simulink model "model31"  (R2024a)
settings: Solver=VariableStepAuto  StartTime=0.0  StopTime=10  MaxStep=1e-3  RelTol=1e-3
values from neighbouring files (symbols this model uses):
  A = [8 1 11 ... (first row only)    [init.m]    (also in init_ex.m)
  B = [-1; -3; 3]    [init.m]    (also in init_ex.m)
  B_f = [1, -1 ... (first row only)    [init.m]    (also in init_ex.m)
  C = [-2 0 -3]    [init.m]    (also in init_ex.m)
  C_st = [0  0 -1 ... (first row only)    [init.m]
  D = 15    [init.m]    (also in init_ex.m)
  D_f = [0 3]    [init.m]    (also in init_ex.m)
  F = G_f - L_st * Y_f    [init.m]
  G = [-5 0 0 ... (first row only)    [init.m]    (also in init_ex.m)
  G_f = [35 10 -28 17 ... (first row only)    [init.m]    (also in init_ex.m)
  G_g = [0 0 0 ... (first row only)    [init.m]    (also in init_ex.m)
  K = [-3.5 1 -3.5]    [init.m]    (also in init_ex.m)
  K_f = [-9.2262   -2.9556    6.9958   -4.9150]    [init.m]    (also in init_ex.m)
  K_g = [0.0703   -0.0562    0.0658]    [init.m]    (also in init_ex.m)
  L_st = -(Y_st * inv(Q_st))'    [init.m]
  Q_inv = inv(Q)    [init.m]    (also in init_ex.m)
  wf0 = [1; 1; 1; 1]    [init.m]    (also in init_ex.m)
  wg0 = [-12; 0; 21]    [init.m]    (also in init_ex.m)
  x0 = [0; 0; 0]    [init.m]    (also in init_ex.m)
  Y = [1; 7; 8]    [init.m]    (also in init_ex.m)
  Y_f = [12 -6 ... (first row only)    [init.m]    (also in init_ex.m)
  Y_g = [1, 1, 0]    [init.m]    (also in init_ex.m)
settings Model: Creator=eva  LastModifiedBy=eva

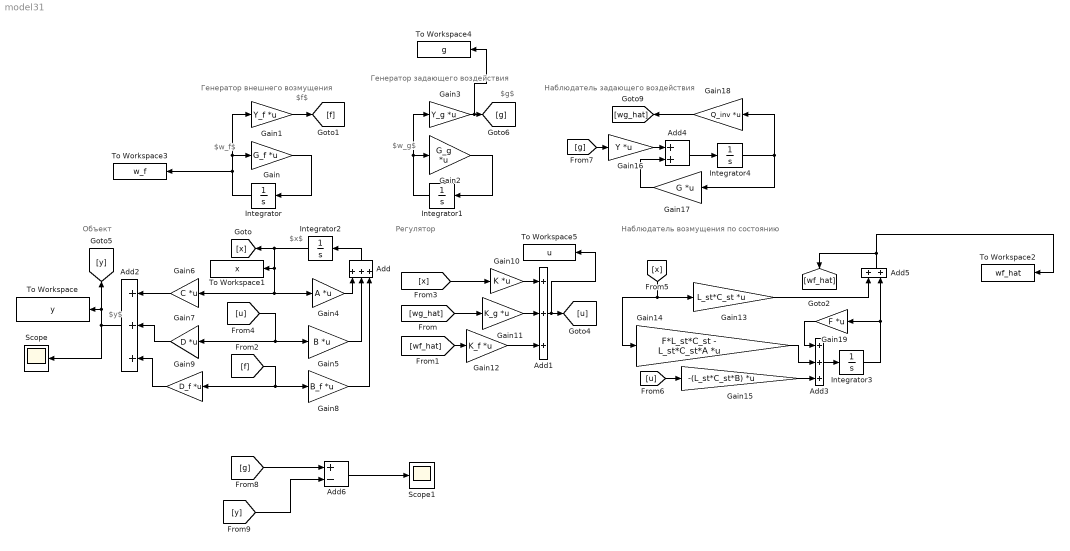
== system model31 ==
  note: Наблюдатель возмущения по состоянию
  note: Объект
  note: Наблюдатель задающего воздействия
  note: $y$
  note: $x$
  note: Регулятор
  note: $g$
  note: $w_f$
  note: Генератор задающего воздействия
  note: $w_g$
  note: $f$
  note: Генератор внешнего возмущения
  Add{,1..3} (4 alike) : Sum  Inputs=+++
  Add4 : Sum
  Add5 : Sum
  Add6 : Sum  Inputs=+-
  Gain : Gain  Gain=G_f  Multiplication=Matrix(K*u)
  Gain1 : Gain  Gain=Y_f  Multiplication=Matrix(K*u)
  Gain10 : Gain  Gain=K  Multiplication=Matrix(K*u)
  Gain11 : Gain  Gain=K_g  Multiplication=Matrix(K*u)
  Gain12 : Gain  Gain=K_f  Multiplication=Matrix(K*u)
  Gain13 : Gain  Gain=L_st*C_st  Multiplication=Matrix(K*u)
  Gain14 : Gain  Gain=F*L_st*C_st - L_st*C_st*A  Multiplication=Matrix(K*u)
  Gain15 : Gain  Gain=-(L_st*C_st*B)  Multiplication=Matrix(K*u)
  Gain16 : Gain  Gain=Y  Multiplication=Matrix(K*u)
  Gain17 : Gain  Gain=G  Multiplication=Matrix(K*u)
  Gain18 : Gain  Gain=Q_inv  Multiplication=Matrix(K*u)
  Gain19 : Gain  Gain=F  Multiplication=Matrix(K*u)
  Gain2 : Gain  Gain=G_g  Multiplication=Matrix(K*u)
  Gain3 : Gain  Gain=Y_g  Multiplication=Matrix(K*u)
  Gain4 : Gain  Gain=A  Multiplication=Matrix(K*u)
  Gain5 : Gain  Gain=B  Multiplication=Matrix(K*u)
  Gain6 : Gain  Gain=C  Multiplication=Matrix(K*u)
  Gain7 : Gain  Gain=D  Multiplication=Matrix(K*u)
  Gain8 : Gain  Gain=B_f  Multiplication=Matrix(K*u)
  Gain9 : Gain  Gain=D_f  Multiplication=Matrix(K*u)
  Integrator : Integrator  InitialCondition=wf0
  Integrator1 : Integrator  InitialCondition=wg0
  Integrator2 : Integrator  InitialCondition=x0
  Integrator3 : Integrator  InitialCondition=[0; 0; 0; 0]
  Integrator4 : Integrator  InitialCondition=[0; 0; 0]
  Scope : Scope
  Scope1 : Scope
  To Workspace : ToWorkspace  VariableName=y  SaveFormat=Structure With Time  SampleTime=-1
  To Workspace1 : ToWorkspace  VariableName=x  SaveFormat=Structure With Time  SampleTime=-1
  To Workspace2 : ToWorkspace  VariableName=wf_hat  SaveFormat=Structure With Time  SampleTime=-1
  To Workspace3 : ToWorkspace  VariableName=w_f  SaveFormat=Structure With Time  SampleTime=-1
  To Workspace4 : ToWorkspace  VariableName=g  SaveFormat=Structure With Time  SampleTime=-1
  To Workspace5 : ToWorkspace  VariableName=u  SaveFormat=Structure With Time  SampleTime=-1
  wires:
  Gain1/1 -> [f]
  Gain2/1 -> Integrator1/1
  Gain4/1 -> Add/1
  Add/1 -> Integrator2/1
  Gain7/1 -> Add2/2
  Gain16/1 -> Add4/1
  Integrator4/1 -> Gain17/1, Gain18/1
  Gain9/1 -> Add2/3
  Integrator/1 -> To Workspace3/1, Gain/1, Gain1/1
  [f] -> Gain8/1, Gain9/1
  [u] -> Gain7/1, Gain5/1
  Gain12/1 -> Add1/3
  Integrator2/1 -> To Workspace1/1, Gain6/1, Gain4/1, [x]
  Gain10/1 -> Add1/1
  Add2/1 -> To Workspace/1, [y], Scope/1
  [wg_hat] -> Gain11/1
  Gain3/1 -> To Workspace4/1, [g]
  Gain8/1 -> Add/3
  Integrator1/1 -> Gain2/1, Gain3/1
  Gain11/1 -> Add1/2
  Gain17/1 -> Add4/2
  [wf_hat] -> Gain12/1
  [g] -> Gain16/1
  Gain18/1 -> [wg_hat]
  Add1/1 -> To Workspace5/1, [u]
  Gain5/1 -> Add/2
  [x] -> Gain10/1
  Add4/1 -> Integrator4/1
  Gain6/1 -> Add2/1
  Gain/1 -> Integrator/1
  [x] -> Gain14/1, Gain13/1
  [u] -> Gain15/1
  Integrator3/1 -> Add5/2, Gain19/1
  Gain13/1 -> Add5/1
  Add5/1 -> To Workspace2/1, [wf_hat]
  Add3/1 -> Integrator3/1
  Gain15/1 -> Add3/3
  Gain14/1 -> Add3/2
  Gain19/1 -> Add3/1
  [g] -> Add6/1
  [y] -> Add6/2
  Add6/1 -> Scope1/1
